simulink model "PositionSensorwithLookUpTable"  (R2023a)
settings: Solver=FixedStepDiscrete  StartTime=0.0  StopTime=10.0  FixedStep=0.005  RelTol=1e-3
model workspace (MAT data in the model file):
  TPSPercent_LkupTbl = Simulink.LookupTable
  TPSPercent_LkupTbl.Table = Simulink.lookuptable.Table
  TPSPercent_LkupTbl.Table.Value = [0 10 20 30 40 50 60 70 80 90 100]
  TPSPercent_LkupTbl.Table.Dimensions = [1 11]
  TPSPercent_LkupTbl.Table.DataType = 'single'
  TPSPercent_LkupTbl.Table.FieldName = 'Table'
  TPSPercent_LkupTbl.Breakpoints = Simulink.lookuptable.Breakpoint
  TPSPercent_LkupTbl.Breakpoints.Value = [0 100 200 300 400 500 600 700 800 900 1000]
  TPSPercent_LkupTbl.Breakpoints.TunableSizeName = 'N1'
  TPSPercent_LkupTbl.Breakpoints.Dimensions = [1 11]
  TPSPercent_LkupTbl.Breakpoints.DataType = 'single'
  TPSPercent_LkupTbl.Breakpoints.FieldName = 'BP1'
  TPSPercent_LkupTbl.AllowMultipleInstancesOfTypeToHaveDifferentTableBreakpointSizes = 0
  TPSPercent_LkupTbl.SupportTunableSize = 0
  TPSPercent_LkupTbl.StructTypeInfo = Simulink.lookuptable.StructTypeInfo
  TPSPercent_LkupTbl.StructTypeInfo.Name = 'MyStruct'
  TPSPercent_LkupTbl.StructTypeInfo.DataScope = 'Auto'
undefined symbols (not defined in the file): TPSPercentBkpt, TPSPercentTbl
settings Model: ParameterArgumentNames=TPSPercent_LkupTbl  Creator=The MathWorks, Inc.  LastModifiedBy=omert
settings SolverCC: AlgebraicLoopSolver=TrustRegion
settings DataIOCC: SaveFormat=StructureWithTime
settings OptimizationCC: DefaultParameterBehavior=Inlined  EnhancedBackFolding=on  PassReuseOutputArgsAs=Individual arguments  ZeroExternalMemoryAtStartup=off  ZeroInternalMemoryAtStartup=off  OptimizeBlockOrder=speed  DifferentSizesBufferReuse=on  OptimizationCustomize=off  EfficientTunableParamExpr=on
settings DebuggingCC: ParameterTunabilityLossMsg=error  UnconnectedInputMsg=warning  UnconnectedOutputMsg=warning  UnconnectedLineMsg=warning
settings ModelReferenceCC: EnableRefExpFcnMdlSchedulingChecks=on
settings SFSimCC: MATLABDynamicMemAlloc=off
settings RTWCC: Description=Embedded Coder  SystemTargetFile=ert.tlc  GenCodeOnly=on  TemplateMakefile=ert_default_tmf  DLArmComputeVersion=19.05
settings CodeAppCC: ForceParamTrailComments=on  IgnoreCustomStorageClasses=off  MaxIdLength=255  OperatorAnnotations=on  SimulinkDataObjDesc=on  SFDataObjDesc=on  InsertBlockDesc=on
settings ERTTargetCC: TargetLangStandard=C99 (ISO)  GenerateSampleERTMain=on  InlinedParameterPlacement=NonHierarchical  ERTCustomFileTemplate=example_file_process.tlc

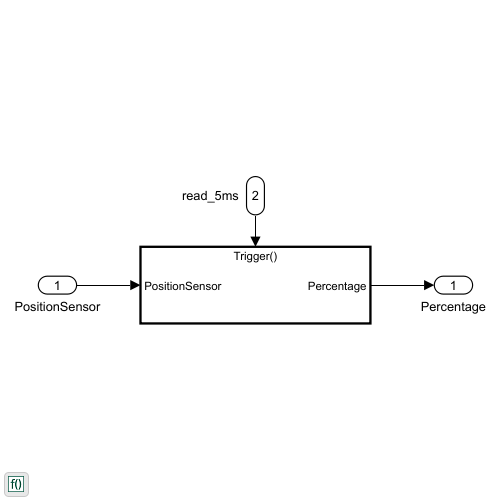
[thumbnail: Simulink's stored preview of the top-level diagram]
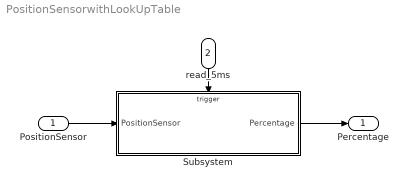
== system PositionSensorwithLookUpTable ==
  PositionSensor : Inport  OutDataTypeStr=uint16  PortDimensions=1
  read_5ms : Inport  Port=2  SampleTime=0.01  OutputFunctionCall=on
  Subsystem : Subsystem
  Percentage : Outport  OutDataTypeStr=single  PortDimensions=1
  wires:
  PositionSensor/1 -> Subsystem/1(PositionSensor)
  Subsystem/1(Percentage) -> Percentage/1
  read_5ms/1 -> Subsystem/Trigger

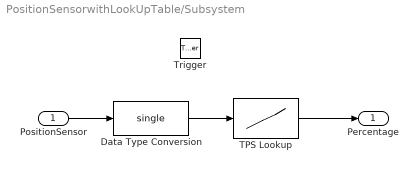
== system PositionSensorwithLookUpTable/Subsystem ==
  PositionSensor : Inport
  Trigger : TriggerPort  TriggerType=function-call  VariantControl=(inherit)  SampleTimeType=periodic  SampleTime=0.005  PortDimensions=1
  Data Type Conversion : DataTypeConversion  OutDataTypeStr=single  SaturateOnIntegerOverflow=off  RndMeth=Floor
  TPS Lookup : Lookup_n-D  NumberOfTableDimensions=1  DataSpecification=Lookup table object  LookupTableObject=TPSPercent_LkupTbl  BreakpointsForDimension1=TPSPercentBkpt  BreakpointsForDimension1DataTypeStr=single  IndexSearchMethod=Linear search  Table=TPSPercentTbl  TableDataTypeStr=single  ExtrapMethod=Clip  InternalRulePriority=Speed  OutDataTypeStr=single  RndMeth=Simplest
  Percentage : Outport
  wires:
  TPS Lookup/1 -> Percentage/1
  PositionSensor/1 -> Data Type Conversion/1
  Data Type Conversion/1 -> TPS Lookup/1
